simulink library "lib_controller"  (R2015a)
settings: Solver=ode45  StartTime=0.0  StopTime=10.0  RelTol=1e-3
values from neighbouring files (symbols this model uses):
  CG_0 = [0,0,0.02]'    [SetupComplete.m]
  g = 9.81    [SetupComplete.m]
  h_M = 0.064    [SetupComplete.m]
  I_BAC_0 = [ Ix,0,Ixz;0,Iy,0;Ixz,0,Iz]    [SetupComplete.m]
  l = 0.3450    (= 0.345)    [NDI_components.m]    (also in SetupComplete.m; robust_controller.m)
  m = 3.51    [SetupComplete.m]
  m_0 = 2.61    [SetupComplete.m]
  m_M = 0.300    (= 0.3)    [SetupComplete.m]
  T_sim = 0.01    [Run3Copter.m]
undefined symbols (not defined in the file or in its folder): Theta_1_roll_last, Theta_2_roll_last, Theta_3_roll_last, V_long_lastA_w_z, V_long_lastAoA, V_roll_last, V_yaw_last, W_long_lastA_w_z, W_long_lastAoA, W_roll_last, W_yaw_last
libraries: simulink x65, Adaptive_FaultTolerantControl x8, lib_controller x5, qcatlib x4, dspinverses x4, aerolibtransform2 x3, aerolib6dofsys x1
(part 4 of 10)

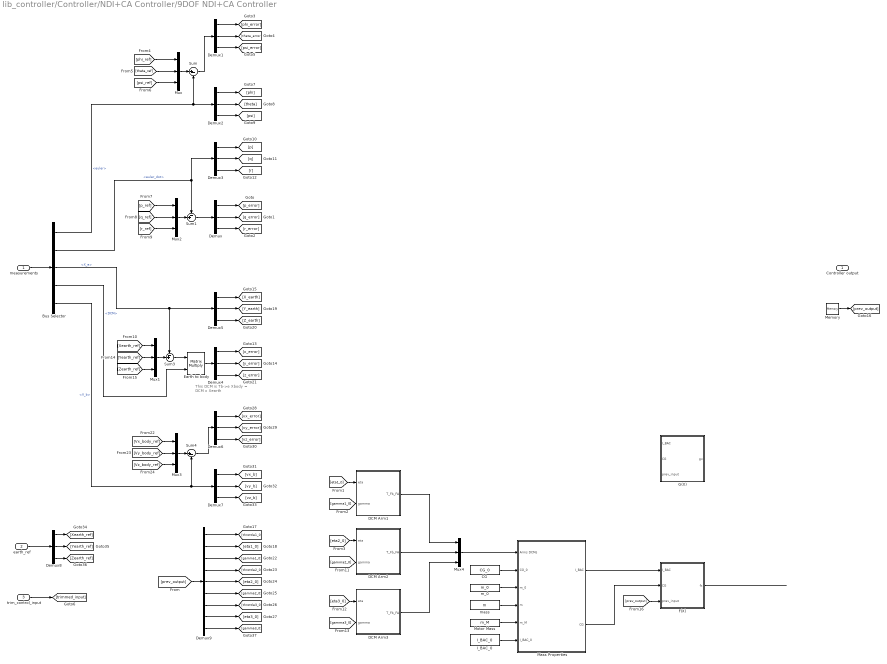
== system lib_controller/Controller/NDI+CA Controller/9DOF NDI+CA Controller ==
  note: This DCM is Tb->e
      | Xbody = DCM x Xearth
  measurements : Inport
  earth_ref : Inport  Port=2
  trim_control_input : Inport  Port=3
  Bus Selector : BusSelector  OutputSignals=euler,euler_dot,X_e,DCM,V_b
  CG : Constant  Value=CG_0
  DCM Arm1 : MATLAB Function  TreatAsAtomicUnit=on
  DCM Arm2 : MATLAB Function  TreatAsAtomicUnit=on
  DCM Arm3 : MATLAB Function  TreatAsAtomicUnit=on
  Demux{,1..8} (9 alike) : Demux  Outputs=3
  Demux9 : Demux  Outputs=9
  Earth to body : Product  Multiplication=Matrix(*)
  F(X) : MATLAB Function  TreatAsAtomicUnit=on
  G(X) : MATLAB Function  TreatAsAtomicUnit=on
  I_BAC_0 : Constant  Value=I_BAC_0
  Mass Properties : Subsystem  TreatAsAtomicUnit=on
  Memory : Memory  LinearizeAsDelay=on
  Motor Mass : Constant  Value=m_M
  Mux{,1..4} (5 alike) : Mux  Inputs=3
  Sum : Sum  Inputs=|+-
  Sum1 : Sum  Inputs=-+|
  Sum3 : Sum  Inputs=-+|
  Sum4 : Sum  Inputs=|+-
  m_0 : Constant  Value=m_0
  mass : Constant  Value=m
  Controller output : Outport
  wires:
  Mux/1 -> Sum/1
  Demux3/3 -> [r]
  Demux3/2 -> [q]
  Demux3/1 -> [p]
  Demux2/1 -> [phi]
  Demux2/2 -> [theta]
  Demux2/3 -> [psi]
  measurements/1 -> Bus Selector/1
  Bus Selector/1 -> Demux2/1, Sum/2  "<euler>"
  Bus Selector/2 -> Demux3/1, Sum1/1  "<euler_dot>"
  Sum1/1 -> Demux/1
  Sum/1 -> Demux1/1
  Demux/3 -> [r_error]
  Demux/2 -> [q_error]
  Demux/1 -> [p_error]
  Demux1/1 -> [phi_error]
  Demux1/2 -> [theta_error]
  Demux1/3 -> [psi_error]
  trim_control_input/1 -> [trimmed_input]
  [theta_ref] -> Mux/2
  [phi_ref] -> Mux/1
  [psi_ref] -> Mux/3
  Mux2/1 -> Sum1/2
  [q_ref] -> Mux2/2
  [p_ref] -> Mux2/1
  [r_ref] -> Mux2/3
  Bus Selector/3 -> Demux5/1, Sum3/1  "<X_e>"
  Demux5/3 -> [Z_earth]
  Demux5/2 -> [Y_earth]
  Demux5/1 -> [X_earth]
  Demux4/3 -> [z_error]
  Demux4/2 -> [y_error]
  Demux4/1 -> [x_error]
  Mux1/1 -> Sum3/2
  [Yearth_ref] -> Mux1/2
  [Xearth_ref] -> Mux1/1
  [Zearth_ref] -> Mux1/3
  Mux3/1 -> Sum4/1
  Demux7/1 -> [vx_b]
  Demux7/2 -> [vy_b]
  Demux7/3 -> [vz_b]
  Bus Selector/5 -> Demux7/1, Sum4/2  "<V_b>"
  Sum4/1 -> Demux6/1
  Demux6/1 -> [vx_error]
  Demux6/2 -> [vy_error]
  Demux6/3 -> [vz_error]
  [Vy_body_ref] -> Mux3/2
  [Vx_body_ref] -> Mux3/1
  [Vz_body_ref] -> Mux3/3
  Bus Selector/4 -> Earth to body/2  "<DCM>"
  Earth to body/1 -> Demux4/1
  Sum3/1 -> Earth to body/1
  Demux8/3 -> [Zearth_ref]
  Demux8/2 -> [Yearth_ref]
  Demux8/1 -> [Xearth_ref]
  earth_ref/1 -> Demux8/1
  ? -> Controller output/1, Memory/1
  Memory/1 -> [prev_output]
  [prev_output] -> Demux9/1
  Demux9/1 -> [throttle1_0]
  Demux9/2 -> [eta1_0]
  Demux9/3 -> [gamma1_0]
  Demux9/4 -> [throttle2_0]
  Demux9/5 -> [eta2_0]
  Demux9/6 -> [gamma2_0]
  Demux9/7 -> [throttle3_0]
  Demux9/8 -> [eta3_0]
  Demux9/9 -> [gamma3_0]
  [eta1_0] -> DCM Arm1/1(eta)
  [gamma1_0] -> DCM Arm1/2(gamma)
  [eta2_0] -> DCM Arm2/1(eta)
  [gamma2_0] -> DCM Arm2/2(gamma)
  [eta3_0] -> DCM Arm3/1(eta)
  [gamma3_0] -> DCM Arm3/2(gamma)
  CG/1 -> Mass Properties/2(CG_0)
  Motor Mass/1 -> Mass Properties/5(m_M)
  I_BAC_0/1 -> Mass Properties/6(I_BAC_0)
  m_0/1 -> Mass Properties/3(m_0)
  mass/1 -> Mass Properties/4(m)
  Mux4/1 -> Mass Properties/1(Arms DCMs)
  DCM Arm1/1(T_Fb_FA) -> Mux4/1
  DCM Arm2/1(T_Fb_FA) -> Mux4/2
  DCM Arm3/1(T_Fb_FA) -> Mux4/3
  Mass Properties/1(I_BAC) -> F(X)/1(I_BAC)
  Mass Properties/2(CG) -> F(X)/2(CG)
  [prev_output] -> F(X)/3(prev_input)
  F(X)/1(fx) -> ?

== system lib_controller/Controller/NDI+CA Controller/ 9DOF NDI+CA Controller - No massic update/1st order reference model ==
  y_ref : Inport
  y_meas : Inport  Port=2
  Bandwidth gain : Gain  Gain=Kb
  Bandwidth gain 1 : Gain  Gain=Kb
  Command FF gain : Gain  Gain=fc
  Command_dot FF gain : Gain  Gain=Kf
  Integral gain : Gain  Gain=fi
  Integrator : Integrator
  Integrator1 : Integrator
  Kref gain : Gain  Gain=Kref
  Sum15 : Sum  Inputs=|+-
  Sum16 : Sum  Inputs=++-
  Sum17 : Sum  Inputs=++|
  Sum5 : Sum  Inputs=|+-
  y_des_dot : Outport
  wires:
  Integral gain/1 -> Integrator1/1
  Bandwidth gain 1/1 -> Integral gain/1
  y_ref/1 -> Sum5/1
  Command_dot FF gain/1 -> Sum17/1
  Command FF gain/1 -> Sum16/1
  Integrator/1 -> Command FF gain/1, Sum15/1, Sum5/2  "y_c"
  y_meas/1 -> Sum16/3, Sum15/2
  Sum16/1 -> Bandwidth gain/1
  Kref gain/1 -> Integrator/1, Command_dot FF gain/1  "y_dot_c"
  Integrator1/1 -> Sum16/2
  Sum17/1 -> y_des_dot/1
  Bandwidth gain/1 -> Sum17/2
  Sum15/1 -> Bandwidth gain 1/1
  Sum5/1 -> Kref gain/1

== system lib_controller/Controller/NDI+CA Controller/ 9DOF NDI+CA Controller - No massic update/9 DOF Ideal (Need more tuning) ==
  note: OUTER POSITION LOOP
  note: Proportional controller around the hovering point. Body rates will be very similar to euler rates.
  note: INNER RATE LOOP TUNING
  note: OUTER ANGLE LOOP TUNING
  note: INNER SPEED LOOP
  Constant{40,55,57,60,62} (5 alike) : Constant
  Constant41 : Constant  Commented=on
  Constant42 : Constant  Commented=on
  Constant43 : Constant  Value=3
  Constant44 : Constant  Value=0
  Constant45 : Constant  Value=0.5
  Constant46 : Constant  Value=0
  Constant47 : Constant  Value=3
  Constant48 : Constant  Value=0
  Constant49 : Constant  Commented=on  Value=0.1
  Constant{50,59,61,63} (4 alike) : Constant  Value=0.2
  Constant51 : Constant  Commented=on  Value=0
  Constant52 : Constant  Commented=on
  Constant53 : Constant  Commented=on  Value=0
  Constant54 : Constant  Value=0.1
  Constant56 : Constant  Value=0.1
  Constant58 : Constant  Value=4
  From38 : From  Commented=on  GotoTag=z_error
  From39 : From  Commented=on  GotoTag=y_error
  From40 : From  Commented=on  GotoTag=x_error
  Goto73 : Goto  Commented=on  GotoTag=Vz_body_ref
  Goto79 : Goto  Commented=on  GotoTag=Vy_body_ref
  Goto80 : Goto  Commented=on  GotoTag=Vx_body_ref
  PID Controller{12,14..16,18..22} (9 alike) : simulink/Continuous/PID Controller  Controller=PI  TimeDomain=Continuous-time  SampleTime=-1  IntegratorMethod=Forward Euler  FilterMethod=Forward Euler  Form=Parallel  UseFilter=on  ControllerParametersSource=external  P=1  I=1  D=0  N=100  InitialConditionSource=internal  InitialConditionForIntegrator=0  InitialConditionForFilter=0  ExternalReset=none  LimitOutput=off  UpperSaturationLimit=inf  LowerSaturationLimit=-inf  LinearizeAsGain=on  AntiWindupMode=none  Kb=1  TrackingMode=off  Kt=1  PParamMin=[]  PParamMax=[]  IParamMin=[]  IParamMax=[]  DParamMin=[]  DParamMax=[]  NParamMin=[]  NParamMax=[]  KbParamMin=[]  KbParamMax=[]  KtParamMin=[]  KtParamMax=[]  POutMin=[]  POutMax=[]  IOutMin=[]  IOutMax=[]  DOutMin=[]  DOutMax=[]  NOutMin=[]  NOutMax=[]  KbOutMin=[]  KbOutMax=[]  KtOutMin=[]  KtOutMax=[]  IntegratorOutMin=[]  IntegratorOutMax=[]  FilterOutMin=[]  FilterOutMax=[]  SumOutMin=[]  SumOutMax=[]  SumI1OutMin=[]  SumI1OutMax=[]  SumI2OutMin=[]  SumI2OutMax=[]  SumI3OutMin=[]  SumI3OutMax=[]  SumDOutMin=[]  SumDOutMax=[]  SaturationOutMin=[]  SaturationOutMax=[]  IntegratorContinuousStateAttributes=''  IntegratorStateMustResolveToSignalObject=off  IntegratorRTWStateStorageClass=Auto  FilterContinuousStateAttributes=''  FilterStateMustResolveToSignalObject=off  FilterRTWStateStorageClass=Auto  DifferentiatorICPrevScaledInput=0  DifferentiatorOutMin=[]  DifferentiatorOutMax=[]
  PID Controller13 : simulink/Continuous/PID Controller  Commented=on  Controller=PI  TimeDomain=Continuous-time  SampleTime=-1  IntegratorMethod=Forward Euler  FilterMethod=Forward Euler  Form=Parallel  UseFilter=on  ControllerParametersSource=external  P=1  I=1  D=0  N=100  InitialConditionSource=internal  InitialConditionForIntegrator=0  InitialConditionForFilter=0  ExternalReset=none  LimitOutput=off  UpperSaturationLimit=inf  LowerSaturationLimit=-inf  LinearizeAsGain=on  AntiWindupMode=none  Kb=1  TrackingMode=off  Kt=1  PParamMin=[]  PParamMax=[]  IParamMin=[]  IParamMax=[]  DParamMin=[]  DParamMax=[]  NParamMin=[]  NParamMax=[]  KbParamMin=[]  KbParamMax=[]  KtParamMin=[]  KtParamMax=[]  POutMin=[]  POutMax=[]  IOutMin=[]  IOutMax=[]  DOutMin=[]  DOutMax=[]  NOutMin=[]  NOutMax=[]  KbOutMin=[]  KbOutMax=[]  KtOutMin=[]  KtOutMax=[]  IntegratorOutMin=[]  IntegratorOutMax=[]  FilterOutMin=[]  FilterOutMax=[]  SumOutMin=[]  SumOutMax=[]  SumI1OutMin=[]  SumI1OutMax=[]  SumI2OutMin=[]  SumI2OutMax=[]  SumI3OutMin=[]  SumI3OutMax=[]  SumDOutMin=[]  SumDOutMax=[]  SaturationOutMin=[]  SaturationOutMax=[]  IntegratorContinuousStateAttributes=''  IntegratorStateMustResolveToSignalObject=off  IntegratorRTWStateStorageClass=Auto  FilterContinuousStateAttributes=''  FilterStateMustResolveToSignalObject=off  FilterRTWStateStorageClass=Auto  DifferentiatorICPrevScaledInput=0  DifferentiatorOutMin=[]  DifferentiatorOutMax=[]
  PID Controller17 : simulink/Continuous/PID Controller  Commented=on  Controller=PI  TimeDomain=Continuous-time  SampleTime=-1  IntegratorMethod=Forward Euler  FilterMethod=Forward Euler  Form=Parallel  UseFilter=on  ControllerParametersSource=external  P=1  I=1  D=0  N=100  InitialConditionSource=internal  InitialConditionForIntegrator=0  InitialConditionForFilter=0  ExternalReset=none  LimitOutput=off  UpperSaturationLimit=inf  LowerSaturationLimit=-inf  LinearizeAsGain=on  AntiWindupMode=none  Kb=1  TrackingMode=off  Kt=1  PParamMin=[]  PParamMax=[]  IParamMin=[]  IParamMax=[]  DParamMin=[]  DParamMax=[]  NParamMin=[]  NParamMax=[]  KbParamMin=[]  KbParamMax=[]  KtParamMin=[]  KtParamMax=[]  POutMin=[]  POutMax=[]  IOutMin=[]  IOutMax=[]  DOutMin=[]  DOutMax=[]  NOutMin=[]  NOutMax=[]  KbOutMin=[]  KbOutMax=[]  KtOutMin=[]  KtOutMax=[]  IntegratorOutMin=[]  IntegratorOutMax=[]  FilterOutMin=[]  FilterOutMax=[]  SumOutMin=[]  SumOutMax=[]  SumI1OutMin=[]  SumI1OutMax=[]  SumI2OutMin=[]  SumI2OutMax=[]  SumI3OutMin=[]  SumI3OutMax=[]  SumDOutMin=[]  SumDOutMax=[]  SaturationOutMin=[]  SaturationOutMax=[]  IntegratorContinuousStateAttributes=''  IntegratorStateMustResolveToSignalObject=off  IntegratorRTWStateStorageClass=Auto  FilterContinuousStateAttributes=''  FilterStateMustResolveToSignalObject=off  FilterRTWStateStorageClass=Auto  DifferentiatorICPrevScaledInput=0  DifferentiatorOutMin=[]  DifferentiatorOutMax=[]
  PID Controller23 : simulink/Continuous/PID Controller  Commented=on  Controller=PI  TimeDomain=Continuous-time  SampleTime=-1  IntegratorMethod=Forward Euler  FilterMethod=Forward Euler  Form=Parallel  UseFilter=on  ControllerParametersSource=external  P=1  I=1  D=0  N=100  InitialConditionSource=internal  InitialConditionForIntegrator=0  InitialConditionForFilter=0  ExternalReset=none  LimitOutput=off  UpperSaturationLimit=inf  LowerSaturationLimit=-inf  LinearizeAsGain=on  AntiWindupMode=none  Kb=1  TrackingMode=off  Kt=1  PParamMin=[]  PParamMax=[]  IParamMin=[]  IParamMax=[]  DParamMin=[]  DParamMax=[]  NParamMin=[]  NParamMax=[]  KbParamMin=[]  KbParamMax=[]  KtParamMin=[]  KtParamMax=[]  POutMin=[]  POutMax=[]  IOutMin=[]  IOutMax=[]  DOutMin=[]  DOutMax=[]  NOutMin=[]  NOutMax=[]  KbOutMin=[]  KbOutMax=[]  KtOutMin=[]  KtOutMax=[]  IntegratorOutMin=[]  IntegratorOutMax=[]  FilterOutMin=[]  FilterOutMax=[]  SumOutMin=[]  SumOutMax=[]  SumI1OutMin=[]  SumI1OutMax=[]  SumI2OutMin=[]  SumI2OutMax=[]  SumI3OutMin=[]  SumI3OutMax=[]  SumDOutMin=[]  SumDOutMax=[]  SaturationOutMin=[]  SaturationOutMax=[]  IntegratorContinuousStateAttributes=''  IntegratorStateMustResolveToSignalObject=off  IntegratorRTWStateStorageClass=Auto  FilterContinuousStateAttributes=''  FilterStateMustResolveToSignalObject=off  FilterRTWStateStorageClass=Auto  DifferentiatorICPrevScaledInput=0  DifferentiatorOutMin=[]  DifferentiatorOutMax=[]
  Sum{17,19..23,26..28} (9 alike) : Sum  Inputs=|++
  Sum18 : Sum  Commented=on  Inputs=|++
  Sum24 : Sum  Commented=on  Inputs=|++
  Sum25 : Sum  Commented=on  Inputs=|++
  Tuning perturbation{12,19..20,22} (4 alike) : Step  Commented=on  Time=20  After=3*pi/180  SampleTime=0
  Tuning perturbation{13..17,23} (6 alike) : Step  Commented=on  Time=20  SampleTime=0
  Tuning perturbation18 : Step  Commented=on  Time=20  After=-3*pi/180  SampleTime=0
  Tuning perturbation21 : Step  Commented=on  Time=20  After=-3*pi/180  SampleTime=0
  wires:
  Constant62/1 -> PID Controller18/2
  [vz_error] -> Sum26/1
  From38/1 -> Sum24/1
  Constant40/1 -> PID Controller12/2
  PID Controller14/1 -> [accY_des]
  [vy_error] -> Sum22/1
  Constant60/1 -> PID Controller19/2
  PID Controller15/1 -> [accX_des]
  Constant41/1 -> PID Controller13/2
  Sum23/1 -> PID Controller15/1
  Sum17/1 -> PID Controller19/1
  Constant49/1 -> PID Controller13/3
  Constant53/1 -> PID Controller23/3
  Sum18/1 -> PID Controller23/1
  Constant58/1 -> PID Controller16/2
  Tuning perturbation16/1 -> Sum25/2
  [psi_error] -> Sum17/1
  Tuning perturbation19/1 -> Sum17/2
  Sum26/1 -> PID Controller16/1
  From39/1 -> Sum25/1
  Tuning perturbation14/1 -> Sum22/2
  PID Controller13/1 -> Goto73/1
  Constant54/1 -> PID Controller14/3
  [q_error] -> Sum20/1
  Tuning perturbation23/1 -> Sum18/2
  Constant52/1 -> PID Controller23/2
  Sum20/1 -> PID Controller21/1
  From40/1 -> Sum18/1
  Tuning perturbation18/1 -> Sum19/2
  Constant61/1 -> PID Controller18/3
  Constant50/1 -> PID Controller16/3
  Tuning perturbation12/1 -> Sum28/2
  Constant44/1 -> PID Controller22/3
  Constant46/1 -> PID Controller21/3
  Tuning perturbation15/1 -> Sum23/2
  Tuning perturbation22/1 -> Sum27/2
  PID Controller12/1 -> [p_ref]
  Sum21/1 -> PID Controller20/1
  Constant43/1 -> PID Controller20/2
  Sum25/1 -> PID Controller17/1
  PID Controller18/1 -> [q_ref]
  Tuning perturbation13/1 -> Sum24/2
  Sum27/1 -> PID Controller22/1
  Constant56/1 -> PID Controller15/3
  Sum19/1 -> PID Controller18/1
  PID Controller23/1 -> Goto80/1
  Sum24/1 -> PID Controller13/1
  PID Controller17/1 -> Goto79/1
  PID Controller20/1 -> [p_dot_des]
  [r_error] -> Sum27/1
  [phi_error] -> Sum28/1
  [vx_error] -> Sum23/1
  PID Controller16/1 -> [accZ_des]
  Sum28/1 -> PID Controller12/1
  Constant47/1 -> PID Controller21/2
  [p_error] -> Sum21/1
  Sum22/1 -> PID Controller14/1
  Tuning perturbation17/1 -> Sum26/2
  Constant63/1 -> PID Controller12/3
  PID Controller21/1 -> [q_dot_des]
  Constant51/1 -> PID Controller17/3
  Tuning perturbation21/1 -> Sum20/2
  Constant45/1 -> PID Controller22/2
  Constant42/1 -> PID Controller17/2
  PID Controller19/1 -> [r_ref]
  Constant59/1 -> PID Controller19/3
  Constant55/1 -> PID Controller14/2
  [theta_error] -> Sum19/1
  PID Controller22/1 -> [r_dot_des]
  Tuning perturbation20/1 -> Sum21/2
  Constant57/1 -> PID Controller15/2
  Constant48/1 -> PID Controller20/3

== system lib_controller/Controller/NDI+CA Controller/ 9DOF NDI+CA Controller - No massic update/Control Allocation 9DOF ==
  Pseudocontrol input : Inport
  Effectiveness control matrix : Inport  Port=2
  Control Allocation 9DOF : Subsystem  VariantControl=(default)
  Pseudoinverse 9DOF : Subsystem  VariantControl=Variant1
  Control output : Outport

== system lib_controller/Controller/NDI+CA Controller/4DOF ANN+NDI+CA Controller - No massic update/Adaptive NN ==
  Model Reference Vars : Inport
  System State Vars : Inport  Port=2
  v_ad^ prev : Inport  Port=3
  Crossed NN : Subsystem  VariantControl=NN on AoA
  v_ad^ : Outport

== system lib_controller/Controller/NDI+CA Controller/4DOF ANN+NDI+CA Controller - No massic update/Adaptive NN1 ==
  Model Reference Vars : Inport
  System State Vars : Inport  Port=2
  v_ad^ prev : Inport  Port=3
  Complete crossed On-line (adaptive) multi-layer NN: AoA : Subsystem  VariantControl=NN on AoA
  v_ad^ : Outport

== system lib_controller/Controller/NDI+CA Controller/4DOF ANN+NDI+CA Controller - No massic update/Control Allocation 4DOF ==
  Pseudocontrol input : Inport
  Effectiveness control matrix : Inport  Port=2
  Control Allocation 4DOF : Subsystem  VariantControl=(default)
  Pseudoinverse : Subsystem  VariantControl=Variant1
  Control output : Outport

== system lib_controller/Controller/NDI+CA Controller/4DOF ANN+NDI+CA Controller - No massic update/On-line (adaptive) multi-layer NNs ==
  v_ad^ prev : Inport
  All_meas : Inport  Port=2
  NN variables : Inport  Port=3
  Bus Selector : BusSelector  OutputSignals=p_chanel_vars,Long chanel,beta_r_chanel
  Long_learning rate : Constant  Value=30.5  SampleTime=T_sim
  Long_reg param : Constant  SampleTime=T_sim
  Mux : Mux  Inputs=3
  Pitch Channel : Subsystem  Variant=on  OverrideUsingVariant=Long HL NN A_w_z
  Roll Channel : Subsystem  Variant=on  OverrideUsingVariant=Roll 1HL NN
  Roll_learning rate : Constant  Value=73  SampleTime=T_sim
  Roll_reg param : Constant  SampleTime=T_sim
  Selector : Selector  InputPortWidth=3
  Selector1 : Selector  InputPortWidth=3  Indices=2
  Selector2 : Selector  InputPortWidth=3  Indices=3
  Yaw Channel : Subsystem  Variant=on  OverrideUsingVariant=Yaw HL NN
  Yaw_learning rate : Constant  Value=20.8  SampleTime=T_sim
  Yaw_reg param : Constant  Value=0.8  SampleTime=T_sim
  v_ad^ prev1 : InportShadow
  v_ad^ prev2 : InportShadow
  v_ad^ : Outport
  wires:
  NN variables/1 -> Bus Selector/1
  Bus Selector/1 -> Roll Channel/2(p_chanel vars)  "<p_chanel_vars>"
  All_meas/1 -> Yaw Channel/3(All_meas), Pitch Channel/3(All_meas), Roll Channel/3(All_meas)
  Roll Channel/1(v_ad_comp) -> Mux/1
  Mux/1 -> v_ad^/1
  v_ad^ prev/1 -> Selector/1
  Selector/1 -> Roll Channel/1(v_ad^ prev)
  Roll_learning rate/1 -> Roll Channel/4(Roll_learning rate)
  Roll_reg param/1 -> Roll Channel/5(Roll reg param)
  Selector1/1 -> Pitch Channel/1(v_ad^ prev)
  Long_learning rate/1 -> Pitch Channel/4(Long_learning rate)
  Long_reg param/1 -> Pitch Channel/5(Long reg param)
  v_ad^ prev1/1 -> Selector1/1
  Bus Selector/2 -> Pitch Channel/2(Long_chanel vars)  "<Long chanel>"
  Yaw_learning rate/1 -> Yaw Channel/4(Yaw_learning rate)
  Yaw_reg param/1 -> Yaw Channel/5(Yaw reg param)
  v_ad^ prev2/1 -> Selector2/1
  Selector2/1 -> Yaw Channel/1(v_ad^ prev)
  Bus Selector/3 -> Yaw Channel/2(Yaw_chanel vars)  "<beta_r_chanel>"
  Yaw Channel/1(v_ad_comp) -> Mux/3
  Pitch Channel/1(v_ad_comp) -> Mux/2

== system lib_controller/Controller/NDI+CA Controller/4DOF ANN+NDI+CA Controller - No massic update/Phi Model Reference ==
  u_ref : Inport
  y_dot : Inport  Port=2
  y : Inport  Port=3
  A_error_dynamics : Constant  Value=[0, 1; -(r*omega_n)^2, -2*xi*(r*omega_n)]
  Bus Creator : BusCreator  Inputs=8
  Kd_y_dot : Gain  Gain=2*xi*(r*omega_n)
  Kp_y : Gain  Gain=(r*omega_n)^2
  P_error_dynamics : Constant  Value=[((r*omega_n)^2+1)/(2*xi*(r*omega_n)) + 2*xi*(r*omega_n)/(r*omega_n)^2, 1/(r*omega_n)^2; 1/(r*omega_n)^2, (1+1/(r*omega_n)^2)/(2*xi*(r*omega_n))]
  Reference Model1 : Adaptive_FaultTolerantControl/Ref Model and P Controller/Reference Model  omega_n=omega_n  xi=xi
  Sum19 : Sum  Inputs=|+-
  Sum20 : Sum  Inputs=+++
  Sum21 : Sum  Inputs=|+-
  b_error_dynamics : Constant  Value=[0; 1]  VectorParams1D=off
  y_dot_dot_des : Outport
  NN_variables : Outport  Port=2
  wires:
  Reference Model1/1 -> Bus Creator/5, Sum20/1  "y_dot_dot_c"
  Reference Model1/3 -> Bus Creator/3, Sum19/1  "y_c"
  u_ref/1 -> Reference Model1/1
  y/1 -> Sum19/2
  Sum19/1 -> Bus Creator/1, Kp_y/1  "y_error"
  Reference Model1/2 -> Bus Creator/4, Sum21/1  "y_dot_c"
  y_dot/1 -> Sum21/2
  Sum21/1 -> Bus Creator/2, Kd_y_dot/1  "y_dot_error"
  Kp_y/1 -> Sum20/3
  Kd_y_dot/1 -> Sum20/2
  Sum20/1 -> y_dot_dot_des/1
  Bus Creator/1 -> NN_variables/1
  P_error_dynamics/1 -> Bus Creator/6  "P_error_dyn"
  A_error_dynamics/1 -> Bus Creator/7  "A_error_dyn"
  b_error_dynamics/1 -> Bus Creator/8  "b_error_dyn"

== system lib_controller/Controller/NDI+CA Controller/4DOF ANN+NDI+CA Controller - No massic update/Psi Model Reference ==
  u_ref : Inport
  y_dot : Inport  Port=2
  A_error_dynamics : Constant  Value=-r/tau
  Bus Creator : BusCreator  Inputs=6
  Kp_y : Gain  Gain=r/tau
  P_error_dynamics : Constant  Value=tau/r
  Reference Model : Adaptive_FaultTolerantControl/Ref Model and P Controller/Reference Model  omega_n=omega_n  xi=xi
  Sum17 : Sum  Inputs=++|
  Sum22 : Sum  Inputs=|+-
  b_error_dynamics : Constant  Value=[1]  VectorParams1D=off
  y_dot_des : Outport
  NN_variables : Outport  Port=2
  wires:
  u_ref/1 -> Reference Model/1
  Reference Model/2 -> Bus Creator/2, Sum22/1  "y_c"
  Reference Model/1 -> Bus Creator/3, Sum17/1  "y_dot_c"
  y_dot/1 -> Sum22/2
  Sum22/1 -> Bus Creator/1, Kp_y/1  "y_error"
  Kp_y/1 -> Sum17/2
  Sum17/1 -> y_dot_des/1
  Bus Creator/1 -> NN_variables/1
  A_error_dynamics/1 -> Bus Creator/5  "A_error_dyn"
  P_error_dynamics/1 -> Bus Creator/4  "P_error_dyn"
  b_error_dynamics/1 -> Bus Creator/6  "b_error_dyn"

== system lib_controller/Controller/NDI+CA Controller/4DOF ANN+NDI+CA Controller - No massic update/Sigmoid  ==
  In : Inport
  Display : Display
  Fcn1 : Fcn  Commented=on  Expr=2.0 ./ (1.0 + exp(-u(4)*u(1:3)))-1
  MATLAB Function : MATLAB Function  TreatAsAtomicUnit=on
  a : Constant  Value=a
  Out : Outport
  wires:
  MATLAB Function/1(y) -> Display/1, Out/1
  In/1 -> MATLAB Function/1(u)
  a/1 -> MATLAB Function/2(a)

== system lib_controller/Controller/NDI+CA Controller/4DOF ANN+NDI+CA Controller - No massic update/Theta Model Reference1 ==
  u_ref : Inport
  y_dot : Inport  Port=2
  y : Inport  Port=3
  A_error_dynamics1 : Constant  Value=[0, 1; -(r*omega_n)^2, -2*xi*(r*omega_n)]
  Bus Creator : BusCreator  Inputs=8
  Kd_y_dot : Gain  Gain=2*xi*(r*omega_n)
  Kp_y : Gain  Gain=(r*omega_n)^2
  P_error_dynamics1 : Constant  Value=[((r*omega_n)^2+1)/(2*xi*(r*omega_n)) + 2*xi*(r*omega_n)/(r*omega_n)^2, 1/(r*omega_n)^2; 1/(r*omega_n)^2, (1+1/(r*omega_n)^2)/(2*xi*(r*omega_n))]
  Reference Model1 : Adaptive_FaultTolerantControl/Ref Model and P Controller/Reference Model  omega_n=omega_n  xi=xi
  Sum19 : Sum  Inputs=|+-
  Sum20 : Sum  Inputs=+++
  Sum21 : Sum  Inputs=|+-
  b_error_dynamics : Constant  Value=[0; 1]  VectorParams1D=off
  y_dot_dot_des : Outport
  NN_variables : Outport  Port=2
  wires:
  b_error_dynamics/1 -> Bus Creator/8  "b_error_dyn"
  A_error_dynamics1/1 -> Bus Creator/7  "A_error_dyn"
  P_error_dynamics1/1 -> Bus Creator/6  "P_error_dyn"
  Bus Creator/1 -> NN_variables/1
  Sum20/1 -> y_dot_dot_des/1
  Kd_y_dot/1 -> Sum20/2
  Kp_y/1 -> Sum20/3
  Sum21/1 -> Bus Creator/2, Kd_y_dot/1  "y_dot_error"
  y_dot/1 -> Sum21/2
  Reference Model1/2 -> Sum21/1, Bus Creator/4  "y_dot_c"
  Sum19/1 -> Kp_y/1, Bus Creator/1  "y_error"
  y/1 -> Sum19/2
  u_ref/1 -> Reference Model1/1
  Reference Model1/3 -> Sum19/1, Bus Creator/3  "y_c"
  Reference Model1/1 -> Sum20/1, Bus Creator/5  "y_dot_dot_c"

== system lib_controller/Controller/NDI+CA Controller/4DOF ANN+NDI+CA Controller - No massic update/Vz_body Model Reference ==
  u_ref : Inport
  y_dot : Inport  Port=2
  A_error_dynamics : Constant  Value=-r/tau
  Bus Creator : BusCreator  Inputs=6
  Kp_y : Gain  Gain=r/tau
  P_error_dynamics : Constant  Value=tau/r
  Reference Model : Adaptive_FaultTolerantControl/Ref Model and P Controller/Reference Model  omega_n=omega_n  xi=xi
  Sum17 : Sum  Inputs=++|
  Sum22 : Sum  Inputs=|+-
  b_error_dynamics : Constant  Value=[1]  VectorParams1D=off
  y_dot_des : Outport
  NN_variables : Outport  Port=2
  wires:
  b_error_dynamics/1 -> Bus Creator/6  "b_error_dyn"
  P_error_dynamics/1 -> Bus Creator/4  "P_error_dyn"
  A_error_dynamics/1 -> Bus Creator/5  "A_error_dyn"
  Bus Creator/1 -> NN_variables/1
  Sum17/1 -> y_dot_des/1
  Kp_y/1 -> Sum17/2
  Sum22/1 -> Kp_y/1, Bus Creator/1  "y_error"
  y_dot/1 -> Sum22/2
  Reference Model/1 -> Sum17/1, Bus Creator/3  "y_dot_c"
  Reference Model/2 -> Sum22/1, Bus Creator/2  "y_c"
  u_ref/1 -> Reference Model/1

== system lib_controller/Controller/NDI+CA Controller/4DOF NDI+CA Controller - No massic update/1st order reference model ==
  y_ref : Inport
  y_meas : Inport  Port=2
  Bandwidth gain : Gain  Gain=Kb
  Bandwidth gain 1 : Gain  Gain=Kb
  Command FF gain : Gain  Gain=fc
  Command_dot FF gain : Gain  Gain=Kf
  Integral gain : Gain  Gain=fi
  Integrator : Integrator
  Integrator1 : Integrator
  Kref gain : Gain  Gain=Kref
  Sum15 : Sum  Inputs=|+-
  Sum16 : Sum  Inputs=++-
  Sum17 : Sum  Inputs=++|
  Sum5 : Sum  Inputs=|+-
  y_des_dot : Outport
  wires:
  Integral gain/1 -> Integrator1/1
  Bandwidth gain 1/1 -> Integral gain/1
  y_ref/1 -> Sum5/1
  Command_dot FF gain/1 -> Sum17/1
  Command FF gain/1 -> Sum16/1
  Integrator/1 -> Command FF gain/1, Sum15/1, Sum5/2  "y_c"
  y_meas/1 -> Sum16/3, Sum15/2
  Sum16/1 -> Bandwidth gain/1
  Kref gain/1 -> Integrator/1, Command_dot FF gain/1  "y_dot_c"
  Integrator1/1 -> Sum16/2
  Sum17/1 -> y_des_dot/1
  Bandwidth gain/1 -> Sum17/2
  Sum15/1 -> Bandwidth gain 1/1
  Sum5/1 -> Kref gain/1

== system lib_controller/Controller/NDI+CA Controller/4DOF NDI+CA Controller - No massic update/1st order reference model2 ==
  y_ref : Inport
  y_meas : Inport  Port=2
  Bandwidth gain : Gain  Gain=Kb
  Bandwidth gain 1 : Gain  Gain=Kb
  Command FF gain : Gain  Gain=fc
  Command_dot FF gain : Gain  Gain=Kf
  Integral gain : Gain  Gain=fi
  Integrator : Integrator
  Integrator1 : Integrator
  Kref gain : Gain  Gain=Kref
  Sum15 : Sum  Inputs=|+-
  Sum16 : Sum  Inputs=++-
  Sum17 : Sum  Inputs=++|
  Sum5 : Sum  Inputs=|+-
  y_des_dot : Outport
  wires:
  Integral gain/1 -> Integrator1/1
  Bandwidth gain 1/1 -> Integral gain/1
  y_ref/1 -> Sum5/1
  Command_dot FF gain/1 -> Sum17/1
  Command FF gain/1 -> Sum16/1
  Integrator/1 -> Command FF gain/1, Sum15/1, Sum5/2  "y_c"
  y_meas/1 -> Sum16/3, Sum15/2
  Sum16/1 -> Bandwidth gain/1
  Kref gain/1 -> Integrator/1, Command_dot FF gain/1  "y_dot_c"
  Integrator1/1 -> Sum16/2
  Sum17/1 -> y_des_dot/1
  Bandwidth gain/1 -> Sum17/2
  Sum15/1 -> Bandwidth gain 1/1
  Sum5/1 -> Kref gain/1

== system lib_controller/Controller/NDI+CA Controller/4DOF NDI+CA Controller - No massic update/1st order reference model3 ==
  y_ref : Inport
  y_meas : Inport  Port=2
  Bandwidth gain : Gain  Gain=Kb
  Bandwidth gain 1 : Gain  Gain=Kb
  Command FF gain : Gain  Gain=fc
  Command_dot FF gain : Gain  Gain=Kf
  Integral gain : Gain  Gain=fi
  Integrator : Integrator
  Integrator1 : Integrator
  Kref gain : Gain  Gain=Kref
  Sum15 : Sum  Inputs=|+-
  Sum16 : Sum  Inputs=++-
  Sum17 : Sum  Inputs=++|
  Sum5 : Sum  Inputs=|+-
  y_des_dot : Outport
  wires:
  Sum5/1 -> Kref gain/1
  Sum15/1 -> Bandwidth gain 1/1
  Bandwidth gain/1 -> Sum17/2
  Sum17/1 -> y_des_dot/1
  Integrator1/1 -> Sum16/2
  Kref gain/1 -> Command_dot FF gain/1, Integrator/1  "y_dot_c"
  Sum16/1 -> Bandwidth gain/1
  y_meas/1 -> Sum15/2, Sum16/3
  Integrator/1 -> Sum5/2, Sum15/1, Command FF gain/1  "y_c"
  Command FF gain/1 -> Sum16/1
  Command_dot FF gain/1 -> Sum17/1
  y_ref/1 -> Sum5/1
  Bandwidth gain 1/1 -> Integral gain/1
  Integral gain/1 -> Integrator1/1

== system lib_controller/Controller/NDI+CA Controller/4DOF NDI+CA Controller - No massic update/Control Allocation 4DOF ==
  Pseudocontrol input : Inport
  Effectiveness control matrix : Inport  Port=2
  Control Allocation 4DOF : Subsystem  VariantControl=(default)
  Pseudoinverse : Subsystem  VariantControl=Variant1
  Control output : Outport

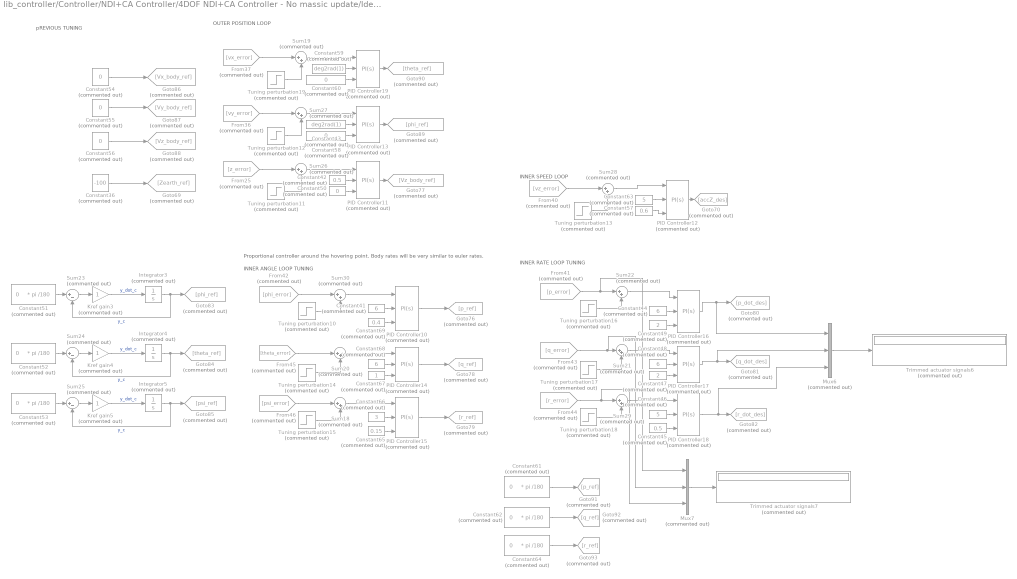
== system lib_controller/Controller/NDI+CA Controller/4DOF NDI+CA Controller - No massic update/Ideal 4DOF controller ==
  note: OUTER POSITION LOOP
  note: Proportional controller around the hovering point. Body rates will be very similar to euler rates.
  note: INNER RATE LOOP TUNING
  note: INNER ANGLE LOOP TUNING
  note: INNER SPEED LOOP
  note: pREVIOUS TUNING
  Constant36 : Constant  Commented=on  Value=-100
  Constant{41,44,48,68} (4 alike) : Constant  Commented=on  Value=6
  Constant42 : Constant  Commented=on  Value=0.5
  Constant43 : Constant  Commented=on  Value=deg2rad(1)
  Constant45 : Constant  Commented=on  Value=0.5
  Constant46 : Constant  Commented=on  Value=5
  Constant47 : Constant  Commented=on  Value=2
  Constant49 : Constant  Commented=on  Value=2
  Constant{50,54..56,58,60} (6 alike) : Constant  Commented=on  Value=0
  Constant{51..53,61..62,64} (6 alike) : Constant  Commented=on  Value="0     * pi /180"
  Constant57 : Constant  Commented=on  Value=0.6
  Constant59 : Constant  Commented=on  Value=deg2rad(1)
  Constant63 : Constant  Commented=on  Value=5
  Constant65 : Constant  Commented=on  Value=0.15
  Constant66 : Constant  Commented=on  Value=3
  Constant67 : Constant  Commented=on
  Constant69 : Constant  Commented=on  Value=0.4
  From25 : From  Commented=on  GotoTag=z_error
  From36 : From  Commented=on  GotoTag=vy_error
  From37 : From  Commented=on  GotoTag=vx_error
  From40 : From  Commented=on  GotoTag=vz_error
  From41 : From  Commented=on  GotoTag=p_error
  From42 : From  Commented=on  GotoTag=phi_error
  From43 : From  Commented=on  GotoTag=q_error
  From44 : From  Commented=on  GotoTag=r_error
  From45 : From  Commented=on  GotoTag=theta_error
  From46 : From  Commented=on  GotoTag=psi_error
  Goto69 : Goto  Commented=on  GotoTag=Zearth_ref
  Goto70 : Goto  Commented=on  GotoTag=accZ_des
  Goto76 : Goto  Commented=on  GotoTag=p_ref
  Goto77 : Goto  Commented=on  GotoTag=Vz_body_ref
  Goto78 : Goto  Commented=on  GotoTag=q_ref
  Goto79 : Goto  Commented=on  GotoTag=r_ref
  Goto80 : Goto  Commented=on  GotoTag=p_dot_des
  Goto81 : Goto  Commented=on  GotoTag=q_dot_des
  Goto82 : Goto  Commented=on  GotoTag=r_dot_des
  Goto83 : Goto  Commented=on  GotoTag=phi_ref
  Goto84 : Goto  Commented=on  GotoTag=theta_ref
  Goto85 : Goto  Commented=on  GotoTag=psi_ref
  Goto86 : Goto  Commented=on  GotoTag=Vx_body_ref
  Goto87 : Goto  Commented=on  GotoTag=Vy_body_ref
  Goto88 : Goto  Commented=on  GotoTag=Vz_body_ref
  Goto89 : Goto  Commented=on  GotoTag=phi_ref
  Goto90 : Goto  Commented=on  GotoTag=theta_ref
  Goto91 : Goto  Commented=on  GotoTag=p_ref
  Goto92 : Goto  Commented=on  GotoTag=q_ref
  Goto93 : Goto  Commented=on  GotoTag=r_ref
  Integrator3 : Integrator  Commented=on
  Integrator4 : Integrator  Commented=on
  Integrator5 : Integrator  Commented=on
  Kref gain3 : Gain  Commented=on
  Kref gain4 : Gain  Commented=on
  Kref gain5 : Gain  Commented=on
  Mux6 : Mux  Commented=on  Inputs=3
  Mux7 : Mux  Commented=on  Inputs=3
  PID Controller{10..15,18..19} (8 alike) : simulink/Continuous/PID Controller  Commented=on  Controller=PI  TimeDomain=Continuous-time  SampleTime=-1  IntegratorMethod=Forward Euler  FilterMethod=Forward Euler  Form=Parallel  UseFilter=on  ControllerParametersSource=external  P=1  I=1  D=0  N=100  InitialConditionSource=internal  InitialConditionForIntegrator=0  InitialConditionForFilter=0  ExternalReset=none  LimitOutput=off  UpperSaturationLimit=inf  LowerSaturationLimit=-inf  LinearizeAsGain=on  AntiWindupMode=none  Kb=1  TrackingMode=off  Kt=1  PParamMin=[]  PParamMax=[]  IParamMin=[]  IParamMax=[]  DParamMin=[]  DParamMax=[]  NParamMin=[]  NParamMax=[]  KbParamMin=[]  KbParamMax=[]  KtParamMin=[]  KtParamMax=[]  POutMin=[]  POutMax=[]  IOutMin=[]  IOutMax=[]  DOutMin=[]  DOutMax=[]  NOutMin=[]  NOutMax=[]  KbOutMin=[]  KbOutMax=[]  KtOutMin=[]  KtOutMax=[]  IntegratorOutMin=[]  IntegratorOutMax=[]  FilterOutMin=[]  FilterOutMax=[]  SumOutMin=[]  SumOutMax=[]  SumI1OutMin=[]  SumI1OutMax=[]  SumI2OutMin=[]  SumI2OutMax=[]  SumI3OutMin=[]  SumI3OutMax=[]  SumDOutMin=[]  SumDOutMax=[]  SaturationOutMin=[]  SaturationOutMax=[]  IntegratorContinuousStateAttributes=''  IntegratorStateMustResolveToSignalObject=off  IntegratorRTWStateStorageClass=Auto  FilterContinuousStateAttributes=''  FilterStateMustResolveToSignalObject=off  FilterRTWStateStorageClass=Auto  DifferentiatorICPrevScaledInput=0  DifferentiatorOutMin=[]  DifferentiatorOutMax=[]
  PID Controller16 : simulink/Continuous/PID Controller  Commented=on  Controller=PI  TimeDomain=Continuous-time  SampleTime=-1  IntegratorMethod=Forward Euler  FilterMethod=Forward Euler  Form=Parallel  UseFilter=on  ControllerParametersSource=external  P=121.80671459326  I=327.532586687046  D=0  N=100  InitialConditionSource=internal  InitialConditionForIntegrator=0  InitialConditionForFilter=0  ExternalReset=none  LimitOutput=off  UpperSaturationLimit=inf  LowerSaturationLimit=-inf  LinearizeAsGain=on  AntiWindupMode=none  Kb=1  TrackingMode=off  Kt=1  PParamMin=[]  PParamMax=[]  IParamMin=[]  IParamMax=[]  DParamMin=[]  DParamMax=[]  NParamMin=[]  NParamMax=[]  KbParamMin=[]  KbParamMax=[]  KtParamMin=[]  KtParamMax=[]  POutMin=[]  POutMax=[]  IOutMin=[]  IOutMax=[]  DOutMin=[]  DOutMax=[]  NOutMin=[]  NOutMax=[]  KbOutMin=[]  KbOutMax=[]  KtOutMin=[]  KtOutMax=[]  IntegratorOutMin=[]  IntegratorOutMax=[]  FilterOutMin=[]  FilterOutMax=[]  SumOutMin=[]  SumOutMax=[]  SumI1OutMin=[]  SumI1OutMax=[]  SumI2OutMin=[]  SumI2OutMax=[]  SumI3OutMin=[]  SumI3OutMax=[]  SumDOutMin=[]  SumDOutMax=[]  SaturationOutMin=[]  SaturationOutMax=[]  IntegratorContinuousStateAttributes=''  IntegratorStateMustResolveToSignalObject=off  IntegratorRTWStateStorageClass=Auto  FilterContinuousStateAttributes=''  FilterStateMustResolveToSignalObject=off  FilterRTWStateStorageClass=Auto  DifferentiatorICPrevScaledInput=0  DifferentiatorOutMin=[]  DifferentiatorOutMax=[]
  PID Controller17 : simulink/Continuous/PID Controller  Commented=on  Controller=PI  TimeDomain=Continuous-time  SampleTime=-1  IntegratorMethod=Forward Euler  FilterMethod=Forward Euler  Form=Parallel  UseFilter=on  ControllerParametersSource=external  P=244.169484479421  I=1759.80724182952  D=0  N=100  InitialConditionSource=internal  InitialConditionForIntegrator=0  InitialConditionForFilter=0  ExternalReset=none  LimitOutput=off  UpperSaturationLimit=inf  LowerSaturationLimit=-inf  LinearizeAsGain=on  AntiWindupMode=none  Kb=1  TrackingMode=off  Kt=1  PParamMin=[]  PParamMax=[]  IParamMin=[]  IParamMax=[]  DParamMin=[]  DParamMax=[]  NParamMin=[]  NParamMax=[]  KbParamMin=[]  KbParamMax=[]  KtParamMin=[]  KtParamMax=[]  POutMin=[]  POutMax=[]  IOutMin=[]  IOutMax=[]  DOutMin=[]  DOutMax=[]  NOutMin=[]  NOutMax=[]  KbOutMin=[]  KbOutMax=[]  KtOutMin=[]  KtOutMax=[]  IntegratorOutMin=[]  IntegratorOutMax=[]  FilterOutMin=[]  FilterOutMax=[]  SumOutMin=[]  SumOutMax=[]  SumI1OutMin=[]  SumI1OutMax=[]  SumI2OutMin=[]  SumI2OutMax=[]  SumI3OutMin=[]  SumI3OutMax=[]  SumDOutMin=[]  SumDOutMax=[]  SaturationOutMin=[]  SaturationOutMax=[]  IntegratorContinuousStateAttributes=''  IntegratorStateMustResolveToSignalObject=off  IntegratorRTWStateStorageClass=Auto  FilterContinuousStateAttributes=''  FilterStateMustResolveToSignalObject=off  FilterRTWStateStorageClass=Auto  DifferentiatorICPrevScaledInput=0  DifferentiatorOutMin=[]  DifferentiatorOutMax=[]
  Sum{18..22,26..30} (10 alike) : Sum  Commented=on  Inputs=|++
  Sum23 : Sum  Commented=on  Inputs=|+-
  Sum24 : Sum  Commented=on  Inputs=|+-
  Sum25 : Sum  Commented=on  Inputs=|+-
  Trimmed actuator signals6 : Display  Commented=on
  Trimmed actuator signals7 : Display  Commented=on
  Tuning perturbation{10,15..16,18} (4 alike) : Step  Commented=on  Time=20  After=3*pi/180  SampleTime=0
  Tuning perturbation{11..13,19} (4 alike) : Step  Commented=on  Time=20  SampleTime=0
  Tuning perturbation14 : Step  Commented=on  Time=20  After=-3*pi/180  SampleTime=0
  Tuning perturbation17 : Step  Commented=on  Time=20  After=-3*pi/180  SampleTime=0
  wires:
  From42/1 -> Sum30/1
  Constant56/1 -> Goto88/1
  Constant55/1 -> Goto87/1
  Constant54/1 -> Goto86/1
  PID Controller12/1 -> Goto70/1
  Mux6/1 -> Trimmed actuator signals6/1
  Tuning perturbation17/1 -> Sum21/2
  Constant59/1 -> PID Controller19/2
  PID Controller13/1 -> Goto89/1
  Tuning perturbation12/1 -> Sum27/2
  From36/1 -> Sum27/1
  Sum27/1 -> PID Controller13/1
  Constant58/1 -> PID Controller13/3
  PID Controller16/1 -> Goto80/1, Mux6/1
  Tuning perturbation14/1 -> Sum20/2
  Tuning perturbation10/1 -> Sum30/2
  Tuning perturbation15/1 -> Sum18/2
  Sum20/1 -> PID Controller14/1
  Constant66/1 -> PID Controller15/2
  PID Controller15/1 -> Goto79/1
  PID Controller14/1 -> Goto78/1
  PID Controller10/1 -> Goto76/1
  Tuning perturbation13/1 -> Sum28/2
  From40/1 -> Sum28/1
  Constant52/1 -> Sum24/1
  Constant61/1 -> Goto91/1
  Constant45/1 -> PID Controller18/3
  Constant49/1 -> PID Controller16/3
  Sum25/1 -> Kref gain5/1
  Kref gain5/1 -> Integrator5/1  "y_dot_c"
  From43/1 -> Sum21/1, Mux7/2
  From41/1 -> Sum22/1, Mux7/1
  From46/1 -> Sum18/1
  From45/1 -> Sum20/1
  Sum28/1 -> PID Controller12/1
  Constant57/1 -> PID Controller12/3
  Constant63/1 -> PID Controller12/2
  Constant64/1 -> Goto93/1
  Constant62/1 -> Goto92/1
  Constant42/1 -> PID Controller11/2
  Constant36/1 -> Goto69/1
  Constant44/1 -> PID Controller16/2
  Mux7/1 -> Trimmed actuator signals7/1
  From44/1 -> Sum29/1, Mux7/3
  Constant48/1 -> PID Controller17/2
  Constant46/1 -> PID Controller18/2
  PID Controller18/1 -> Goto82/1, Mux6/3
  PID Controller17/1 -> Goto81/1, Mux6/2
  Integrator3/1 -> Goto83/1, Sum23/2  "y_c"
  Constant51/1 -> Sum23/1
  PID Controller19/1 -> Goto90/1
  Tuning perturbation19/1 -> Sum19/2
  From37/1 -> Sum19/1
  Sum19/1 -> PID Controller19/1
  Constant60/1 -> PID Controller19/3
  Constant43/1 -> PID Controller13/2
  PID Controller11/1 -> Goto77/1
  Tuning perturbation11/1 -> Sum26/2
  From25/1 -> Sum26/1
  Sum26/1 -> PID Controller11/1
  Constant50/1 -> PID Controller11/3
  Integrator5/1 -> Goto85/1, Sum25/2  "y_c"
  Constant53/1 -> Sum25/1
  Sum24/1 -> Kref gain4/1
  Kref gain4/1 -> Integrator4/1  "y_dot_c"
  Sum23/1 -> Kref gain3/1
  Kref gain3/1 -> Integrator3/1  "y_dot_c"
  Tuning perturbation16/1 -> Sum22/2
  Tuning perturbation18/1 -> Sum29/2
  Sum21/1 -> PID Controller17/1
  Sum29/1 -> PID Controller18/1
  Sum22/1 -> PID Controller16/1
  Constant47/1 -> PID Controller17/3
  Sum18/1 -> PID Controller15/1
  Sum30/1 -> PID Controller10/1
  Constant67/1 -> PID Controller14/3
  Constant69/1 -> PID Controller10/3
  Constant41/1 -> PID Controller10/2
  Constant68/1 -> PID Controller14/2
  Constant65/1 -> PID Controller15/3
  Integrator4/1 -> Sum24/2, Goto84/1  "y_c"

== system lib_controller/Controller/NDI+CA Controller/9DOF ANN+NDI+CA Controller - No massic update/Adaptive NN ==
  Model Reference Vars : Inport
  System State Vars : Inport  Port=2
  v_ad^ prev : Inport  Port=3
  Crossed NN : Subsystem  VariantControl=NN on AoA
  v_ad^ : Outport

== system lib_controller/Controller/NDI+CA Controller/9DOF ANN+NDI+CA Controller - No massic update/Control Allocation 9DOF ==
  Pseudocontrol input : Inport
  Effectiveness control matrix : Inport  Port=2
  Control Allocation 9DOF : Subsystem  VariantControl=(default)
  Pseudoinverse 9DOF : Subsystem  VariantControl=Variant1
  Control output : Outport

== system lib_controller/Controller/NDI+CA Controller/9DOF ANN+NDI+CA Controller - No massic update/Psi Model Reference ==
  u_ref : Inport
  y_dot : Inport  Port=2
  A_error_dynamics : Constant  Value=-r/tau
  Bus Creator : BusCreator  Inputs=6
  Kp_y : Gain  Gain=r/tau
  P_error_dynamics : Constant  Value=tau/r
  Reference Model : Adaptive_FaultTolerantControl/Ref Model and P Controller/Reference Model  omega_n=omega_n  xi=xi
  Sum17 : Sum  Inputs=++|
  Sum22 : Sum  Inputs=|+-
  b_error_dynamics : Constant  Value=[1]  VectorParams1D=off
  y_dot_des : Outport
  NN_variables : Outport  Port=2
  wires:
  u_ref/1 -> Reference Model/1
  Reference Model/2 -> Bus Creator/2, Sum22/1  "y_c"
  Reference Model/1 -> Bus Creator/3, Sum17/1  "y_dot_c"
  y_dot/1 -> Sum22/2
  Sum22/1 -> Bus Creator/1, Kp_y/1  "y_error"
  Kp_y/1 -> Sum17/2
  Sum17/1 -> y_dot_des/1
  Bus Creator/1 -> NN_variables/1
  A_error_dynamics/1 -> Bus Creator/5  "A_error_dyn"
  P_error_dynamics/1 -> Bus Creator/4  "P_error_dyn"
  b_error_dynamics/1 -> Bus Creator/6  "b_error_dyn"

== system lib_controller/Controller/NDI+CA Controller/9DOF ANN+NDI+CA Controller - No massic update/Sigmoid  ==
  In : Inport
  Display : Display
  Fcn1 : Fcn  Commented=on  Expr=2.0 ./ (1.0 + exp(-u(4)*u(1:3)))-1
  MATLAB Function : MATLAB Function  TreatAsAtomicUnit=on
  a : Constant  Value=a
  Out : Outport
  wires:
  MATLAB Function/1(y) -> Display/1, Out/1
  In/1 -> MATLAB Function/1(u)
  a/1 -> MATLAB Function/2(a)

== system lib_controller/Controller/NDI+CA Controller/9DOF NDI+CA Controller/Mass Properties ==
  Arms DCMs : Inport
  CG_0 : Inport  Port=2
  m_0 : Inport  Port=3
  m : Inport  Port=4
  m_M : Inport  Port=5
  I_BAC_0 : Inport  Port=6
  Arm Inertia : MATLAB Function  TreatAsAtomicUnit=on
  Bus Selector : BusSelector  OutputSignals=T_FaFb1,T_FaFb2,T_FaFb3
  CG position : Sum
  Divide : Product  Inputs=*/
  Divide1 : Product  Inputs=**
  Divide2 : Product  Inputs=/*
  Divide3 : Product  Inputs=**
  Motors Pos sum : Sum  Inputs=+++
  Total I_BAC : Sum
  I_BAC : Outport
  CG : Outport  Port=2
  wires:
  Arms DCMs/1 -> Bus Selector/1
  Bus Selector/3 -> Arm Inertia/3(T3_FAFb)  "<T_FaFb3>"
  Bus Selector/2 -> Arm Inertia/2(T2_FAFb)  "<T_FaFb2>"
  Bus Selector/1 -> Arm Inertia/1(T1_FAFb)  "<T_FaFb1>"
  Total I_BAC/1 -> I_BAC/1
  m_0/1 -> Divide/1
  m/1 -> Divide/2, Divide2/1
  CG_0/1 -> Divide1/1
  Divide/1 -> Divide1/2
  m_M/1 -> Divide2/2
  CG position/1 -> CG/1
  Divide1/1 -> CG position/1
  Motors Pos sum/1 -> Divide3/1
  Divide2/1 -> Divide3/2
  Divide3/1 -> CG position/2
  Arm Inertia/3(r2_M) -> Motors Pos sum/2
  Arm Inertia/4(r3_M) -> Motors Pos sum/1
  Arm Inertia/1(I_M) -> Total I_BAC/2
  I_BAC_0/1 -> Total I_BAC/1
  Arm Inertia/2(r1_M) -> Motors Pos sum/3

== system lib_controller/Controller/NDI+CA Controller/ 9DOF NDI+CA Controller - No massic update/Control Allocation 9DOF/Control Allocation 9DOF ==
  note: Enabler override saturations and override
      | them with zero to avoid actuators being
      | locked by control allocation algorithm
  note: Weights used to normalize different
      | inputs between controllers.
      | Throttle - 0 to 1
      | Servo - 0 to 2*pi
  note: Position and rate limits for
      | tricopter actuators
  Pseudocontrol input : Inport
  Effectiveness control matrix : Inport  Port=2
  "Control allocator Completed " : qcatlib/Control allocator Completed   alg=WLS  CA_type=QP  iter_max=4  gamma=1e6  k_B=6  m_B=9  T=0.01  tol=0
  Control desired (0 to minimize control effort) : Constant  Value=zeros(1,9)
  Control desired (Timmed 9DOF) : Constant  Value=[0.6049, -0.7465,-0.07355,0.6044,-0.7422,0.4171,0.6044,0.5941,0.417]
  Control positions deviation Weight W1 : Constant  Value=diag(1./[1,2*pi,2*pi,1,2*pi,2*pi,1,2*pi,2*pi] )
  Control rate deviation Weight W2 : Constant  Value=diag(1./[1,2*pi,2*pi,1,2*pi,2*pi,1,2*pi,2*pi] )
  Enalbe/Disable : Constant
  Error Weight Wv2 : Constant  Value=blkdiag(1,1,1, 1/(2*pi), 1/(2*pi), 1/(2*pi))
  Position limits 9DOF : Constant  Value=[ [0,-deg2rad(165),-deg2rad(90),0,-deg2rad(165),-deg2rad(15),0,-deg2rad(165),-deg2rad(90)]', [1,deg2rad(165),deg2rad(15),1,deg2rad(165),deg2rad(90),1,deg2rad(165),deg2rad(15)]']
  Rates limits 9DOF : Constant  Value=[ [-17,-1,-1,-17,-1,-1,-17,-1,-1]', [17,1,1,17,1,1,17,1,1]']*2
  Reshape1 : Reshape  OutputDimensionality=Customize  OutputDimensions=[6,9]
  Reshape2 : Reshape  OutputDimensions=[6,1]
  Terminator : Terminator
  Terminator1 : Terminator
  Unit Delay : UnitDelay  SampleTime=-1
  manual Initial saturations : Constant  Value=zeros(9,1)
  Control output : Outport  PortDimensions=9
  wires:
  "Control allocator Completed "/2 -> Terminator/1
  "Control allocator Completed "/3 -> Terminator1/1
  Effectiveness control matrix/1 -> Reshape1/1
  Reshape1/1 -> "Control allocator Completed "/4
  Position limits 9DOF/1 -> "Control allocator Completed "/5
  Rates limits 9DOF/1 -> "Control allocator Completed "/6
  Error Weight Wv2/1 -> "Control allocator Completed "/7
  Control positions deviation Weight W1/1 -> "Control allocator Completed "/8
  Control rate deviation Weight W2/1 -> "Control allocator Completed "/9
  manual Initial saturations/1 -> "Control allocator Completed "/10
  Enalbe/Disable/1 -> "Control allocator Completed "/11
  Reshape2/1 -> Control output/1
  "Control allocator Completed "/1 -> Reshape2/1, Unit Delay/1
  Unit Delay/1 -> "Control allocator Completed "/2
  Pseudocontrol input/1 -> "Control allocator Completed "/1
  Control desired (Timmed 9DOF)/1 -> "Control allocator Completed "/3

== system lib_controller/Controller/NDI+CA Controller/ 9DOF NDI+CA Controller - No massic update/Control Allocation 9DOF/Pseudoinverse 9DOF ==
  Pseudocontrol input : Inport
  Effectiveness control matrix : Inport  Port=2
  Product1 : Product  Multiplication=Matrix(*)
  Pseudoinverse : dspinverses/Pseudoinverse  wanterr=off
  Reshape1 : Reshape  OutputDimensions=[6,1]
  Control output : Outport  PortDimensions=9
  wires:
  Product1/1 -> Reshape1/1
  Pseudoinverse/1 -> Product1/1
  Effectiveness control matrix/1 -> Pseudoinverse/1
  Pseudocontrol input/1 -> Product1/2
  Reshape1/1 -> Control output/1
